simulink model "newparameterstest"  (R2021a)
settings: Solver=VariableStepAuto  StartTime=0.0  StopTime=2  RelTol=1e-3
undefined symbols (not defined in the file or in its folder): Ion, Lithium
libraries: spsCurrentMeasurementLib x25, spsVoltageMeasurementLib x19, spsSeriesRLCBranchLib x11, spsGroundLib x6, powerlib_extras x5, dspsigops x3, spsPower3phInstantaneousLib x3, eeTotalHarmonicDistorsion x3, spsIGBTDiodeLib x2, spsUniversalBridgeLib x2, spsBatteryLib x1, spsParallelRLCBranchLib x1
(part 2 of 2)

== matlab function newparameterstest/Battery/MATLAB Function ==
  data: discharge input; y output; charge input; soc input; override input; midcontrol input
function y = fcn(discharge,charge,soc,override,midcontrol)

if(soc<8.995 && override==0)
    y = charge;
else
    if(soc<8.995 && override==1)
        y = discharge;
    else
        if(soc>9.005 && override==0)
        y = discharge; 
        else
           if(soc>9.005 && override==1)
             y = charge; 
           else
               if(midcontrol == 0)
                   y =charge;
               else
                   y = discharge;
               end
           end
        end
    end
end
